simulink model "secondorder_mimumumphase_qfilter"  (R2019b)
settings: Solver=FixedStepAuto  StartTime=0.0  StopTime=50  FixedStep=0.001  RelTol=1e-3
values from neighbouring files (symbols this model uses):
  w_c = 5    [design.m]
  wn = 1    [design.m]
  zeta = 0.01    [design.m]
libraries: simulink x1
settings Model: Creator=henry  LastModifiedBy=henry

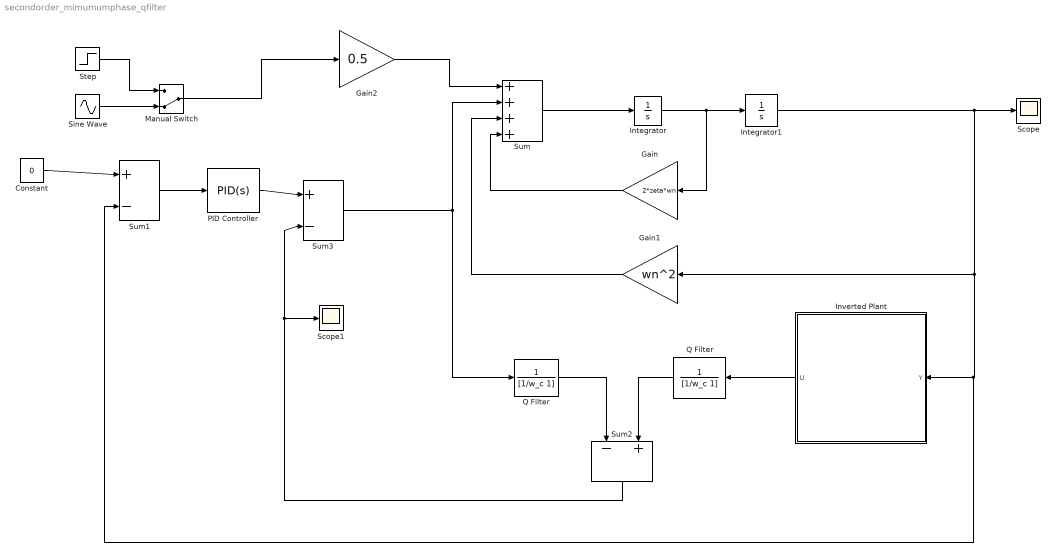
== system secondorder_mimumumphase_qfilter ==
  Constant : Constant  Value=0
  Gain : Gain  Gain=2*zeta*wn
  Gain1 : Gain  Gain=wn^2
  Gain2 : Gain  Gain=0.5
  Integrator : Integrator
  Integrator1 : Integrator  InitialCondition=0.1
  Inverted Plant : Subsystem
  Manual Switch : ManualSwitch  CurrentSetting=0
  PID Controller : simulink/Continuous/PID Controller  Controller=PID  Form=Ideal  TimeDomain=Continuous-time  SampleTime=-1  IntegratorMethod=Forward Euler  FilterMethod=Forward Euler  ControllerParametersSource=internal  P=15  I=7  D=1  UseFilter=on  N=100  TunerSelectOption=Transfer Function Based (PID Tuner App)  InitialConditionSource=internal  InitialConditionForIntegrator=0  InitialConditionForFilter=0  DifferentiatorICPrevScaledInput=0  ExternalReset=none  TrackingMode=off  Kt=1  LimitOutput=off  UpperSaturationLimit=inf  LowerSaturationLimit=-inf  LinearizeAsGain=on  AntiWindupMode=none  Kb=1  POutMin=[]  POutMax=[]  IOutMin=[]  IOutMax=[]  DOutMin=[]  DOutMax=[]  NOutMin=[]  NOutMax=[]  SumOutMin=[]  SumOutMax=[]  SaturationOutMin=[]  SaturationOutMax=[]  PParamMin=[]  PParamMax=[]  IParamMin=[]  IParamMax=[]  DParamMin=[]  DParamMax=[]  NParamMin=[]  NParamMax=[]  KbParamMin=[]  KbParamMax=[]  KtParamMin=[]  KtParamMax=[]  KbOutMin=[]  KbOutMax=[]  KtOutMin=[]  KtOutMax=[]  IntegratorOutMin=[]  IntegratorOutMax=[]  FilterOutMin=[]  FilterOutMax=[]  SumI1OutMin=[]  SumI1OutMax=[]  SumI2OutMin=[]  SumI2OutMax=[]  SumI3OutMin=[]  SumI3OutMax=[]  SumI4OutMin=[]  SumI4OutMax=[]  SumDOutMin=[]  SumDOutMax=[]  DifferentiatorOutMin=[]  DifferentiatorOutMax=[]  FilterDiffOutCoefMin=[]  FilterDiffOutCoefMax=[]  ReciprocalOutMin=[]  ReciprocalOutMax=[]  SumDenOutMin=[]  SumDenOutMax=[]  SumNumOutMin=[]  SumNumOutMax=[]  DivideOutMin=[]  DivideOutMax=[]  IntegratorContinuousStateAttributes=''  IntegratorStateMustResolveToSignalObject=off  IntegratorRTWStateStorageClass=Auto  FilterContinuousStateAttributes=''  FilterStateMustResolveToSignalObject=off  FilterRTWStateStorageClass=Auto  ParallelPVariant=Passthrough  IdealPVariant=InternalParameters  IVariant=InternalParameters  DVariant=InternalParameters  IntegratorVariant=Continuous  SatVariant=Disabled  AWVariant=Passthrough  PCopyVariant=Disabled  TRVariant=Disabled  FdbkBlocksVariant=Forward  IdealPFdbkVariant=Disabled  SatFdbkVariant=Disabled  DerivativeFilterVariant=ContFilter  NVariant=InternalParameters  NCopyVariant=Disabled  FilterICVariant=InternalICsFilter  IntegratorICVariant=InternalICs  ExternalResetVariant=Disabled  TRSumVariant=Passthrough  SumFdbkVariant=Disabled  SumVariant=Sum_PID
  Q Filter : TransferFcn  Numerator=[0 1]  Denominator=[1/w_c 1]
  "Q Filter " : TransferFcn  Numerator=[0 1]  Denominator=[1/w_c 1]
  Scope : Scope
  Scope1 : Scope
  Sine Wave : Sin  Bias=1  SampleTime=0
  Step : Step  SampleTime=0
  Sum : Sum  Inputs=+|+|+|+
  Sum1 : Sum  Inputs=+|-
  Sum2 : Sum  Inputs=-|+
  Sum3 : Sum  Inputs=+|-
  wires:
  Sum/1 -> Integrator/1
  Integrator/1 -> Gain/1, Integrator1/1
  Integrator1/1 -> Gain1/1, Inverted Plant/1(Y), Sum1/2, Scope/1
  Gain/1 -> Sum/4
  Gain1/1 -> Sum/3
  Gain2/1 -> Sum/1
  Sum1/1 -> PID Controller/1
  Constant/1 -> Sum1/1
  Q Filter/1 -> Sum2/1
  Inverted Plant/1(U) -> "Q Filter "/1
  PID Controller/1 -> Sum3/1
  Sum3/1 -> Q Filter/1, Sum/2
  Sum2/1 -> Scope1/1, Sum3/2
  "Q Filter "/1 -> Sum2/2
  Step/1 -> Manual Switch/1
  Sine Wave/1 -> Manual Switch/2
  Manual Switch/1 -> Gain2/1

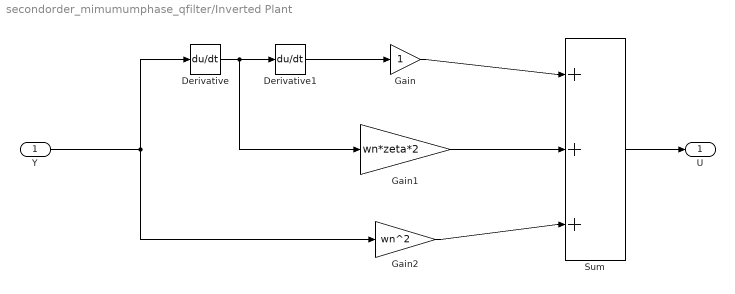
== system secondorder_mimumumphase_qfilter/Inverted Plant ==
  Y : Inport
  Derivative : Derivative
  Derivative1 : Derivative
  Gain : Gain
  Gain1 : Gain  Gain=wn*zeta*2
  Gain2 : Gain  Gain=wn^2
  Sum : Sum  Inputs=+|+|+
  U : Outport
  wires:
  Y/1 -> Gain2/1, Derivative/1
  Derivative1/1 -> Gain/1
  Derivative/1 -> Gain1/1, Derivative1/1
  Gain/1 -> Sum/1
  Gain1/1 -> Sum/2
  Sum/1 -> U/1
  Gain2/1 -> Sum/3
